simulink model "Addzeros"  (R2020a)
settings: Solver=VariableStepAuto  StartTime=0.0  StopTime=10.0  RelTol=1e-3
values from neighbouring files (symbols this model uses):
  K = 1    [main.m]
settings Model: Creator=Kimo Store  LastModifiedBy=Kimo Store

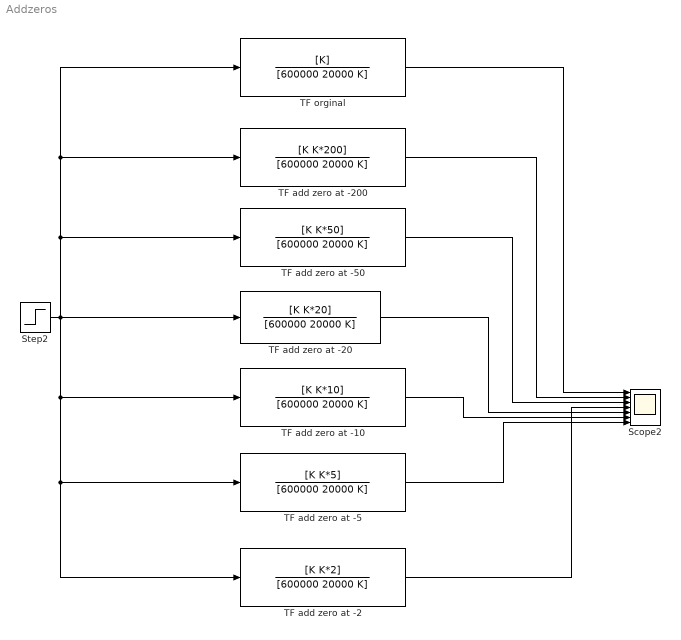
== system Addzeros ==
  Scope2 : Scope  NumInputPorts=7
  Step2 : Step  Time=0  SampleTime=0
  TF add zero at -10 : TransferFcn  Numerator=[K K*10]  Denominator=[600000 20000 K]
  TF add zero at -2 : TransferFcn  Numerator=[K K*2]  Denominator=[600000 20000 K]
  TF add zero at -20 : TransferFcn  Numerator=[K K*20]  Denominator=[600000 20000 K]
  TF add zero at -200 : TransferFcn  Numerator=[K K*200]  Denominator=[600000 20000 K]
  TF add zero at -5 : TransferFcn  Numerator=[K K*5]  Denominator=[600000 20000 K]
  TF add zero at -50 : TransferFcn  Numerator=[K K*50]  Denominator=[600000 20000 K]
  "TF orginal " : TransferFcn  Numerator=[K]  Denominator=[600000 20000 K]
  wires:
  Step2/1 -> TF add zero at -10/1, TF add zero at -5/1, TF add zero at -2/1, TF add zero at -20/1, TF add zero at -200/1, "TF orginal "/1, TF add zero at -50/1
  TF add zero at -20/1 -> Scope2/5
  TF add zero at -5/1 -> Scope2/7
  TF add zero at -50/1 -> Scope2/3
  "TF orginal "/1 -> Scope2/1
  TF add zero at -10/1 -> Scope2/6
  TF add zero at -2/1 -> Scope2/4
  TF add zero at -200/1 -> Scope2/2
